simulink model "hcu_main_dspace"  (Simulink 8.2)
settings: Solver=FixedStepDiscrete  StartTime=0.0  StopTime=Inf  FixedStep=0.005  RelTol=1e-3
PostLoadFcn:
  | , if any(exist('dsrtsu_mdlpostloadfcn', 'file') == [2, 3, 6]), try dsrtsu_mdlpostloadfcn('Execute', bdroot); catch fprintf('Error in PostLoadFcn (dsrtsu_mdlpostloadfcn) for model "%s":\n %s\n', bdroot, lasterr); end, end,
values from neighbouring files (symbols this model uses):
  C_TASK_5MS_S = (	C_TICK_TIME_S      	)    [hcu_local_hdr.m]
  ENUM_GEARPOSN_1ST = uint8(  1  )    [hcu_local_hdr.m]
  ENUM_GEARPOSN_2ND = uint8(  2  )    [hcu_local_hdr.m]
  ENUM_GEARPOSN_3RD = uint8(  3  )    [hcu_local_hdr.m]
  ENUM_GEARPOSN_4TH = uint8(  4  )    [hcu_local_hdr.m]
  ENUM_GEARPOSN_5TH = uint8(  5  )    [hcu_local_hdr.m]
  ENUM_GEARPOSN_6TH = uint8(  6  )    [hcu_local_hdr.m]
  ENUM_GEARPOSN_R = uint8(  7  )    [hcu_local_hdr.m]
undefined symbols (not defined in the file or in its folder): rticanmm_blockfcn, rticanmm_initfcn
libraries: rtimmsu_dsrtlib x3, simulink x2, hal x2, app x1, rtiethernetudplib x1, inp x1, outp x1, hcu_lib x1
(part 3 of 4)

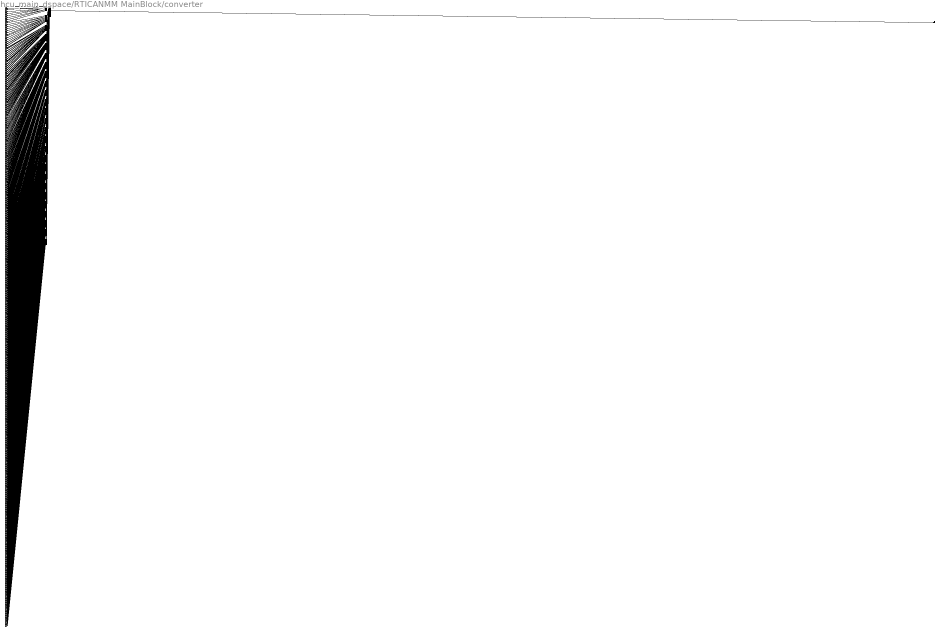
== system hcu_main_dspace/RTICANMM MainBlock/converter ==
  in_1 : Inport
  in_2 : Inport  Port=2
  in_3 : Inport  Port=3
  in_4 : Inport  Port=4
  in_5 : Inport  Port=5
  in_6 : Inport  Port=6
  in_7 : Inport  Port=7
  in_8 : Inport  Port=8
  in_9 : Inport  Port=9
  in_10 : Inport  Port=10
  in_11 : Inport  Port=11
  in_12 : Inport  Port=12
  in_13 : Inport  Port=13
  in_14 : Inport  Port=14
  in_15 : Inport  Port=15
  in_16 : Inport  Port=16
  in_17 : Inport  Port=17
  in_18 : Inport  Port=18
  in_19 : Inport  Port=19
  in_20 : Inport  Port=20
  in_21 : Inport  Port=21
  in_22 : Inport  Port=22
  in_23 : Inport  Port=23
  in_24 : Inport  Port=24
  in_25 : Inport  Port=25
  in_26 : Inport  Port=26
  in_27 : Inport  Port=27
  in_28 : Inport  Port=28
  in_29 : Inport  Port=29
  in_30 : Inport  Port=30
  in_31 : Inport  Port=31
  in_32 : Inport  Port=32
  in_33 : Inport  Port=33
  in_34 : Inport  Port=34
  in_35 : Inport  Port=35
  in_36 : Inport  Port=36
  in_37 : Inport  Port=37
  in_38 : Inport  Port=38
  in_39 : Inport  Port=39
  in_40 : Inport  Port=40
  in_41 : Inport  Port=41
  in_42 : Inport  Port=42
  in_43 : Inport  Port=43
  in_44 : Inport  Port=44
  in_45 : Inport  Port=45
  in_46 : Inport  Port=46
  in_47 : Inport  Port=47
  in_48 : Inport  Port=48
  in_49 : Inport  Port=49
  in_50 : Inport  Port=50
  in_51 : Inport  Port=51
  in_52 : Inport  Port=52
  in_53 : Inport  Port=53
  in_54 : Inport  Port=54
  in_55 : Inport  Port=55
  in_56 : Inport  Port=56
  in_57 : Inport  Port=57
  in_58 : Inport  Port=58
  in_59 : Inport  Port=59
  in_60 : Inport  Port=60
  in_61 : Inport  Port=61
  in_62 : Inport  Port=62
  in_63 : Inport  Port=63
  in_64 : Inport  Port=64
  in_65 : Inport  Port=65
  in_66 : Inport  Port=66
  in_67 : Inport  Port=67
  in_68 : Inport  Port=68
  in_69 : Inport  Port=69
  in_70 : Inport  Port=70
  in_71 : Inport  Port=71
  in_72 : Inport  Port=72
  in_73 : Inport  Port=73
  in_74 : Inport  Port=74
  in_75 : Inport  Port=75
  in_76 : Inport  Port=76
  in_77 : Inport  Port=77
  in_78 : Inport  Port=78
  in_79 : Inport  Port=79
  in_80 : Inport  Port=80
  in_81 : Inport  Port=81
  in_82 : Inport  Port=82
  in_83 : Inport  Port=83
  in_84 : Inport  Port=84
  in_85 : Inport  Port=85
  in_86 : Inport  Port=86
  in_87 : Inport  Port=87
  in_88 : Inport  Port=88
  in_89 : Inport  Port=89
  in_90 : Inport  Port=90
  in_91 : Inport  Port=91
  in_92 : Inport  Port=92
  in_93 : Inport  Port=93
  in_94 : Inport  Port=94
  in_95 : Inport  Port=95
  in_96 : Inport  Port=96
  in_97 : Inport  Port=97
  in_98 : Inport  Port=98
  in_99 : Inport  Port=99
  in_100 : Inport  Port=100
  in_101 : Inport  Port=101
  in_102 : Inport  Port=102
  in_103 : Inport  Port=103
  in_104 : Inport  Port=104
  in_105 : Inport  Port=105
  in_106 : Inport  Port=106
  in_107 : Inport  Port=107
  in_108 : Inport  Port=108
  in_109 : Inport  Port=109
  in_110 : Inport  Port=110
  in_111 : Inport  Port=111
  in_112 : Inport  Port=112
  in_113 : Inport  Port=113
  in_114 : Inport  Port=114
  in_115 : Inport  Port=115
  in_116 : Inport  Port=116
  in_117 : Inport  Port=117
  in_118 : Inport  Port=118
  in_119 : Inport  Port=119
  in_120 : Inport  Port=120
  in_121 : Inport  Port=121
  in_122 : Inport  Port=122
  in_123 : Inport  Port=123
  in_124 : Inport  Port=124
  in_125 : Inport  Port=125
  in_126 : Inport  Port=126
  in_127 : Inport  Port=127
  in_128 : Inport  Port=128
  in_129 : Inport  Port=129
  in_130 : Inport  Port=130
  in_131 : Inport  Port=131
  in_132 : Inport  Port=132
  in_133 : Inport  Port=133
  in_134 : Inport  Port=134
  in_135 : Inport  Port=135
  in_136 : Inport  Port=136
  in_137 : Inport  Port=137
  in_138 : Inport  Port=138
  in_139 : Inport  Port=139
  in_140 : Inport  Port=140
  in_141 : Inport  Port=141
  in_142 : Inport  Port=142
  in_143 : Inport  Port=143
  in_144 : Inport  Port=144
  in_145 : Inport  Port=145
  in_146 : Inport  Port=146
  in_147 : Inport  Port=147
  in_148 : Inport  Port=148
  in_149 : Inport  Port=149
  in_150 : Inport  Port=150
  in_151 : Inport  Port=151
  in_152 : Inport  Port=152
  in_153 : Inport  Port=153
  in_154 : Inport  Port=154
  in_155 : Inport  Port=155
  in_156 : Inport  Port=156
  in_157 : Inport  Port=157
  in_158 : Inport  Port=158
  in_159 : Inport  Port=159
  in_160 : Inport  Port=160
  in_161 : Inport  Port=161
  in_162 : Inport  Port=162
  in_163 : Inport  Port=163
  in_164 : Inport  Port=164
  in_165 : Inport  Port=165
  in_166 : Inport  Port=166
  in_167 : Inport  Port=167
  in_168 : Inport  Port=168
  in_169 : Inport  Port=169
  in_170 : Inport  Port=170
  in_171 : Inport  Port=171
  in_172 : Inport  Port=172
  in_173 : Inport  Port=173
  in_174 : Inport  Port=174
  in_175 : Inport  Port=175
  in_176 : Inport  Port=176
  in_177 : Inport  Port=177
  in_178 : Inport  Port=178
  in_179 : Inport  Port=179
  in_180 : Inport  Port=180
  in_181 : Inport  Port=181
  in_182 : Inport  Port=182
  in_183 : Inport  Port=183
  in_184 : Inport  Port=184
  in_185 : Inport  Port=185
  in_186 : Inport  Port=186
  in_187 : Inport  Port=187
  in_188 : Inport  Port=188
  in_189 : Inport  Port=189
  in_190 : Inport  Port=190
  in_191 : Inport  Port=191
  in_192 : Inport  Port=192
  in_193 : Inport  Port=193
  in_194 : Inport  Port=194
  in_195 : Inport  Port=195
  in_196 : Inport  Port=196
  in_197 : Inport  Port=197
  in_198 : Inport  Port=198
  in_199 : Inport  Port=199
  in_200 : Inport  Port=200
  in_201 : Inport  Port=201
  in_202 : Inport  Port=202
  in_203 : Inport  Port=203
  in_204 : Inport  Port=204
  in_205 : Inport  Port=205
  in_206 : Inport  Port=206
  in_207 : Inport  Port=207
  in_208 : Inport  Port=208
  in_209 : Inport  Port=209
  in_210 : Inport  Port=210
  in_211 : Inport  Port=211
  in_212 : Inport  Port=212
  in_213 : Inport  Port=213
  in_214 : Inport  Port=214
  in_215 : Inport  Port=215
  in_216 : Inport  Port=216
  in_217 : Inport  Port=217
  in_218 : Inport  Port=218
  in_219 : Inport  Port=219
  in_220 : Inport  Port=220
  in_221 : Inport  Port=221
  in_222 : Inport  Port=222
  in_223 : Inport  Port=223
  in_224 : Inport  Port=224
  in_225 : Inport  Port=225
  in_226 : Inport  Port=226
  in_227 : Inport  Port=227
  in_228 : Inport  Port=228
  in_229 : Inport  Port=229
  in_230 : Inport  Port=230
  in_231 : Inport  Port=231
  in_232 : Inport  Port=232
  in_233 : Inport  Port=233
  in_234 : Inport  Port=234
  in_235 : Inport  Port=235
  in_236 : Inport  Port=236
  in_237 : Inport  Port=237
  in_238 : Inport  Port=238
  in_239 : Inport  Port=239
  in_240 : Inport  Port=240
  in_241 : Inport  Port=241
  in_242 : Inport  Port=242
  in_243 : Inport  Port=243
  in_244 : Inport  Port=244
  in_245 : Inport  Port=245
  in_246 : Inport  Port=246
  in_247 : Inport  Port=247
  in_248 : Inport  Port=248
  in_249 : Inport  Port=249
  in_250 : Inport  Port=250
  in_251 : Inport  Port=251
  in_252 : Inport  Port=252
  in_253 : Inport  Port=253
  in_254 : Inport  Port=254
  in_255 : Inport  Port=255
  in_256 : Inport  Port=256
  in_257 : Inport  Port=257
  in_258 : Inport  Port=258
  in_259 : Inport  Port=259
  in_260 : Inport  Port=260
  in_261 : Inport  Port=261
  in_262 : Inport  Port=262
  in_263 : Inport  Port=263
  in_264 : Inport  Port=264
  in_265 : Inport  Port=265
  in_266 : Inport  Port=266
  in_267 : Inport  Port=267
  in_268 : Inport  Port=268
  in_269 : Inport  Port=269
  in_270 : Inport  Port=270
  in_271 : Inport  Port=271
  in_272 : Inport  Port=272
  in_273 : Inport  Port=273
  in_274 : Inport  Port=274
  in_275 : Inport  Port=275
  in_276 : Inport  Port=276
  in_277 : Inport  Port=277
  in_278 : Inport  Port=278
  in_279 : Inport  Port=279
  in_280 : Inport  Port=280
  in_281 : Inport  Port=281
  in_282 : Inport  Port=282
  in_283 : Inport  Port=283
  in_284 : Inport  Port=284
  in_285 : Inport  Port=285
  in_286 : Inport  Port=286
  in_287 : Inport  Port=287
  in_288 : Inport  Port=288
  in_289 : Inport  Port=289
  in_290 : Inport  Port=290
  in_291 : Inport  Port=291
  in_292 : Inport  Port=292
  in_293 : Inport  Port=293
  in_294 : Inport  Port=294
  in_295 : Inport  Port=295
  in_296 : Inport  Port=296
  in_297 : Inport  Port=297
  in_298 : Inport  Port=298
  in_299 : Inport  Port=299
  in_300 : Inport  Port=300
  in_301 : Inport  Port=301
  in_302 : Inport  Port=302
  in_303 : Inport  Port=303
  in_304 : Inport  Port=304
  in_305 : Inport  Port=305
  in_306 : Inport  Port=306
  in_307 : Inport  Port=307
  in_308 : Inport  Port=308
  in_309 : Inport  Port=309
  in_310 : Inport  Port=310
  in_311 : Inport  Port=311
  in_312 : Inport  Port=312
  in_313 : Inport  Port=313
  in_314 : Inport  Port=314
  in_315 : Inport  Port=315
  in_316 : Inport  Port=316
  in_317 : Inport  Port=317
  in_318 : Inport  Port=318
  in_319 : Inport  Port=319
  in_320 : Inport  Port=320
  in_321 : Inport  Port=321
  in_322 : Inport  Port=322
  in_323 : Inport  Port=323
  in_324 : Inport  Port=324
  in_325 : Inport  Port=325
  in_326 : Inport  Port=326
  in_327 : Inport  Port=327
  in_328 : Inport  Port=328
  in_329 : Inport  Port=329
  in_330 : Inport  Port=330
  in_331 : Inport  Port=331
  in_332 : Inport  Port=332
  in_333 : Inport  Port=333
  in_334 : Inport  Port=334
  Lane_Details : BusCreator  Inputs=9
  Mux : BusCreator  Inputs=26
  RTICANMMCaptureMessage_{1..25} (25 alike) : BusCreator  Inputs=13
  out : Outport
  wires:
  in_1/1 -> Lane_Details/1  "Left_Guard_Rail"
  Lane_Details/1 -> Mux/1  "Lane_Details"
  in_2/1 -> Lane_Details/2  "Right_Guard_Rail"
  in_3/1 -> Lane_Details/3  "construction_area"
  in_4/1 -> Lane_Details/4  "Right_LDW_Availability"
  in_5/1 -> Lane_Details/5  "Left_LDW_Availability"
  in_6/1 -> Lane_Details/6  "Yaw_Angle"
  in_7/1 -> Lane_Details/7  "Pitch_Angle"
  in_8/1 -> Lane_Details/8  "Number_of_Lanes"
  in_9/1 -> Lane_Details/9  "Position_in_Lanes"
  in_10/1 -> RTICANMMCaptureMessage_1/1  "Status"
  RTICANMMCaptureMessage_1/1 -> Mux/2  "RTICANMMCaptureMessage_1"
  in_11/1 -> RTICANMMCaptureMessage_1/2  "Time"
  in_12/1 -> RTICANMMCaptureMessage_1/3  "ID"
  in_13/1 -> RTICANMMCaptureMessage_1/4  "MessageIDFormat"
  in_14/1 -> RTICANMMCaptureMessage_1/5  "Length"
  in_15/1 -> RTICANMMCaptureMessage_1/6  "RAW_Byte_1"
  in_16/1 -> RTICANMMCaptureMessage_1/7  "RAW_Byte_2"
  in_17/1 -> RTICANMMCaptureMessage_1/8  "RAW_Byte_3"
  in_18/1 -> RTICANMMCaptureMessage_1/9  "RAW_Byte_4"
  in_19/1 -> RTICANMMCaptureMessage_1/10  "RAW_Byte_5"
  in_20/1 -> RTICANMMCaptureMessage_1/11  "RAW_Byte_6"
  in_21/1 -> RTICANMMCaptureMessage_1/12  "RAW_Byte_7"
  in_22/1 -> RTICANMMCaptureMessage_1/13  "RAW_Byte_8"
  in_23/1 -> RTICANMMCaptureMessage_2/1  "Status"
  RTICANMMCaptureMessage_2/1 -> Mux/3  "RTICANMMCaptureMessage_2"
  in_24/1 -> RTICANMMCaptureMessage_2/2  "Time"
  in_25/1 -> RTICANMMCaptureMessage_2/3  "ID"
  in_26/1 -> RTICANMMCaptureMessage_2/4  "MessageIDFormat"
  in_27/1 -> RTICANMMCaptureMessage_2/5  "Length"
  in_28/1 -> RTICANMMCaptureMessage_2/6  "RAW_Byte_1"
  in_29/1 -> RTICANMMCaptureMessage_2/7  "RAW_Byte_2"
  in_30/1 -> RTICANMMCaptureMessage_2/8  "RAW_Byte_3"
  in_31/1 -> RTICANMMCaptureMessage_2/9  "RAW_Byte_4"
  in_32/1 -> RTICANMMCaptureMessage_2/10  "RAW_Byte_5"
  in_33/1 -> RTICANMMCaptureMessage_2/11  "RAW_Byte_6"
  in_34/1 -> RTICANMMCaptureMessage_2/12  "RAW_Byte_7"
  in_35/1 -> RTICANMMCaptureMessage_2/13  "RAW_Byte_8"
  in_36/1 -> RTICANMMCaptureMessage_3/1  "Status"
  RTICANMMCaptureMessage_3/1 -> Mux/4  "RTICANMMCaptureMessage_3"
  in_37/1 -> RTICANMMCaptureMessage_3/2  "Time"
  in_38/1 -> RTICANMMCaptureMessage_3/3  "ID"
  in_39/1 -> RTICANMMCaptureMessage_3/4  "MessageIDFormat"
  in_40/1 -> RTICANMMCaptureMessage_3/5  "Length"
  in_41/1 -> RTICANMMCaptureMessage_3/6  "RAW_Byte_1"
  in_42/1 -> RTICANMMCaptureMessage_3/7  "RAW_Byte_2"
  in_43/1 -> RTICANMMCaptureMessage_3/8  "RAW_Byte_3"
  in_44/1 -> RTICANMMCaptureMessage_3/9  "RAW_Byte_4"
  in_45/1 -> RTICANMMCaptureMessage_3/10  "RAW_Byte_5"
  in_46/1 -> RTICANMMCaptureMessage_3/11  "RAW_Byte_6"
  in_47/1 -> RTICANMMCaptureMessage_3/12  "RAW_Byte_7"
  in_48/1 -> RTICANMMCaptureMessage_3/13  "RAW_Byte_8"
  in_49/1 -> RTICANMMCaptureMessage_4/1  "Status"
  RTICANMMCaptureMessage_4/1 -> Mux/5  "RTICANMMCaptureMessage_4"
  in_50/1 -> RTICANMMCaptureMessage_4/2  "Time"
  in_51/1 -> RTICANMMCaptureMessage_4/3  "ID"
  in_52/1 -> RTICANMMCaptureMessage_4/4  "MessageIDFormat"
  in_53/1 -> RTICANMMCaptureMessage_4/5  "Length"
  in_54/1 -> RTICANMMCaptureMessage_4/6  "RAW_Byte_1"
  in_55/1 -> RTICANMMCaptureMessage_4/7  "RAW_Byte_2"
  in_56/1 -> RTICANMMCaptureMessage_4/8  "RAW_Byte_3"
  in_57/1 -> RTICANMMCaptureMessage_4/9  "RAW_Byte_4"
  in_58/1 -> RTICANMMCaptureMessage_4/10  "RAW_Byte_5"
  in_59/1 -> RTICANMMCaptureMessage_4/11  "RAW_Byte_6"
  in_60/1 -> RTICANMMCaptureMessage_4/12  "RAW_Byte_7"
  in_61/1 -> RTICANMMCaptureMessage_4/13  "RAW_Byte_8"
  in_62/1 -> RTICANMMCaptureMessage_5/1  "Status"
  RTICANMMCaptureMessage_5/1 -> Mux/6  "RTICANMMCaptureMessage_5"
  in_63/1 -> RTICANMMCaptureMessage_5/2  "Time"
  in_64/1 -> RTICANMMCaptureMessage_5/3  "ID"
  in_65/1 -> RTICANMMCaptureMessage_5/4  "MessageIDFormat"
  in_66/1 -> RTICANMMCaptureMessage_5/5  "Length"
  in_67/1 -> RTICANMMCaptureMessage_5/6  "RAW_Byte_1"
  in_68/1 -> RTICANMMCaptureMessage_5/7  "RAW_Byte_2"
  in_69/1 -> RTICANMMCaptureMessage_5/8  "RAW_Byte_3"
  in_70/1 -> RTICANMMCaptureMessage_5/9  "RAW_Byte_4"
  in_71/1 -> RTICANMMCaptureMessage_5/10  "RAW_Byte_5"
  in_72/1 -> RTICANMMCaptureMessage_5/11  "RAW_Byte_6"
  in_73/1 -> RTICANMMCaptureMessage_5/12  "RAW_Byte_7"
  in_74/1 -> RTICANMMCaptureMessage_5/13  "RAW_Byte_8"
  in_75/1 -> RTICANMMCaptureMessage_6/1  "Status"
  RTICANMMCaptureMessage_6/1 -> Mux/7  "RTICANMMCaptureMessage_6"
  in_76/1 -> RTICANMMCaptureMessage_6/2  "Time"
  in_77/1 -> RTICANMMCaptureMessage_6/3  "ID"
  in_78/1 -> RTICANMMCaptureMessage_6/4  "MessageIDFormat"
  in_79/1 -> RTICANMMCaptureMessage_6/5  "Length"
  in_80/1 -> RTICANMMCaptureMessage_6/6  "RAW_Byte_1"
  in_81/1 -> RTICANMMCaptureMessage_6/7  "RAW_Byte_2"
  in_82/1 -> RTICANMMCaptureMessage_6/8  "RAW_Byte_3"
  in_83/1 -> RTICANMMCaptureMessage_6/9  "RAW_Byte_4"
  in_84/1 -> RTICANMMCaptureMessage_6/10  "RAW_Byte_5"
  in_85/1 -> RTICANMMCaptureMessage_6/11  "RAW_Byte_6"
  in_86/1 -> RTICANMMCaptureMessage_6/12  "RAW_Byte_7"
  in_87/1 -> RTICANMMCaptureMessage_6/13  "RAW_Byte_8"
  in_88/1 -> RTICANMMCaptureMessage_7/1  "Status"
  RTICANMMCaptureMessage_7/1 -> Mux/8  "RTICANMMCaptureMessage_7"
  in_89/1 -> RTICANMMCaptureMessage_7/2  "Time"
  in_90/1 -> RTICANMMCaptureMessage_7/3  "ID"
  in_91/1 -> RTICANMMCaptureMessage_7/4  "MessageIDFormat"
  in_92/1 -> RTICANMMCaptureMessage_7/5  "Length"
  in_93/1 -> RTICANMMCaptureMessage_7/6  "RAW_Byte_1"
  in_94/1 -> RTICANMMCaptureMessage_7/7  "RAW_Byte_2"
  in_95/1 -> RTICANMMCaptureMessage_7/8  "RAW_Byte_3"
  in_96/1 -> RTICANMMCaptureMessage_7/9  "RAW_Byte_4"
  in_97/1 -> RTICANMMCaptureMessage_7/10  "RAW_Byte_5"
  in_98/1 -> RTICANMMCaptureMessage_7/11  "RAW_Byte_6"
  in_99/1 -> RTICANMMCaptureMessage_7/12  "RAW_Byte_7"
  in_100/1 -> RTICANMMCaptureMessage_7/13  "RAW_Byte_8"
  in_101/1 -> RTICANMMCaptureMessage_8/1  "Status"
  RTICANMMCaptureMessage_8/1 -> Mux/9  "RTICANMMCaptureMessage_8"
  in_102/1 -> RTICANMMCaptureMessage_8/2  "Time"
  in_103/1 -> RTICANMMCaptureMessage_8/3  "ID"
  in_104/1 -> RTICANMMCaptureMessage_8/4  "MessageIDFormat"
  in_105/1 -> RTICANMMCaptureMessage_8/5  "Length"
  in_106/1 -> RTICANMMCaptureMessage_8/6  "RAW_Byte_1"
  in_107/1 -> RTICANMMCaptureMessage_8/7  "RAW_Byte_2"
  in_108/1 -> RTICANMMCaptureMessage_8/8  "RAW_Byte_3"
  in_109/1 -> RTICANMMCaptureMessage_8/9  "RAW_Byte_4"
  in_110/1 -> RTICANMMCaptureMessage_8/10  "RAW_Byte_5"
  in_111/1 -> RTICANMMCaptureMessage_8/11  "RAW_Byte_6"
  in_112/1 -> RTICANMMCaptureMessage_8/12  "RAW_Byte_7"
  in_113/1 -> RTICANMMCaptureMessage_8/13  "RAW_Byte_8"
  in_114/1 -> RTICANMMCaptureMessage_9/1  "Status"
  RTICANMMCaptureMessage_9/1 -> Mux/10  "RTICANMMCaptureMessage_9"
  in_115/1 -> RTICANMMCaptureMessage_9/2  "Time"
  in_116/1 -> RTICANMMCaptureMessage_9/3  "ID"
  in_117/1 -> RTICANMMCaptureMessage_9/4  "MessageIDFormat"
  in_118/1 -> RTICANMMCaptureMessage_9/5  "Length"
  in_119/1 -> RTICANMMCaptureMessage_9/6  "RAW_Byte_1"
  in_120/1 -> RTICANMMCaptureMessage_9/7  "RAW_Byte_2"
  in_121/1 -> RTICANMMCaptureMessage_9/8  "RAW_Byte_3"
  in_122/1 -> RTICANMMCaptureMessage_9/9  "RAW_Byte_4"
  in_123/1 -> RTICANMMCaptureMessage_9/10  "RAW_Byte_5"
  in_124/1 -> RTICANMMCaptureMessage_9/11  "RAW_Byte_6"
  in_125/1 -> RTICANMMCaptureMessage_9/12  "RAW_Byte_7"
  in_126/1 -> RTICANMMCaptureMessage_9/13  "RAW_Byte_8"
  in_127/1 -> RTICANMMCaptureMessage_10/1  "Status"
  RTICANMMCaptureMessage_10/1 -> Mux/11  "RTICANMMCaptureMessage_10"
  in_128/1 -> RTICANMMCaptureMessage_10/2  "Time"
  in_129/1 -> RTICANMMCaptureMessage_10/3  "ID"
  in_130/1 -> RTICANMMCaptureMessage_10/4  "MessageIDFormat"
  in_131/1 -> RTICANMMCaptureMessage_10/5  "Length"
  in_132/1 -> RTICANMMCaptureMessage_10/6  "RAW_Byte_1"
  in_133/1 -> RTICANMMCaptureMessage_10/7  "RAW_Byte_2"
  in_134/1 -> RTICANMMCaptureMessage_10/8  "RAW_Byte_3"
  in_135/1 -> RTICANMMCaptureMessage_10/9  "RAW_Byte_4"
  in_136/1 -> RTICANMMCaptureMessage_10/10  "RAW_Byte_5"
  in_137/1 -> RTICANMMCaptureMessage_10/11  "RAW_Byte_6"
  in_138/1 -> RTICANMMCaptureMessage_10/12  "RAW_Byte_7"
  in_139/1 -> RTICANMMCaptureMessage_10/13  "RAW_Byte_8"
  in_140/1 -> RTICANMMCaptureMessage_11/1  "Status"
  RTICANMMCaptureMessage_11/1 -> Mux/12  "RTICANMMCaptureMessage_11"
  in_141/1 -> RTICANMMCaptureMessage_11/2  "Time"
  in_142/1 -> RTICANMMCaptureMessage_11/3  "ID"
  in_143/1 -> RTICANMMCaptureMessage_11/4  "MessageIDFormat"
  in_144/1 -> RTICANMMCaptureMessage_11/5  "Length"
  in_145/1 -> RTICANMMCaptureMessage_11/6  "RAW_Byte_1"
  in_146/1 -> RTICANMMCaptureMessage_11/7  "RAW_Byte_2"
  in_147/1 -> RTICANMMCaptureMessage_11/8  "RAW_Byte_3"
  in_148/1 -> RTICANMMCaptureMessage_11/9  "RAW_Byte_4"
  in_149/1 -> RTICANMMCaptureMessage_11/10  "RAW_Byte_5"
  in_150/1 -> RTICANMMCaptureMessage_11/11  "RAW_Byte_6"
  in_151/1 -> RTICANMMCaptureMessage_11/12  "RAW_Byte_7"
  in_152/1 -> RTICANMMCaptureMessage_11/13  "RAW_Byte_8"
  in_153/1 -> RTICANMMCaptureMessage_12/1  "Status"
  RTICANMMCaptureMessage_12/1 -> Mux/13  "RTICANMMCaptureMessage_12"
  in_154/1 -> RTICANMMCaptureMessage_12/2  "Time"
  in_155/1 -> RTICANMMCaptureMessage_12/3  "ID"
  in_156/1 -> RTICANMMCaptureMessage_12/4  "MessageIDFormat"
  in_157/1 -> RTICANMMCaptureMessage_12/5  "Length"
  in_158/1 -> RTICANMMCaptureMessage_12/6  "RAW_Byte_1"
  in_159/1 -> RTICANMMCaptureMessage_12/7  "RAW_Byte_2"
  in_160/1 -> RTICANMMCaptureMessage_12/8  "RAW_Byte_3"
  in_161/1 -> RTICANMMCaptureMessage_12/9  "RAW_Byte_4"
  in_162/1 -> RTICANMMCaptureMessage_12/10  "RAW_Byte_5"
  in_163/1 -> RTICANMMCaptureMessage_12/11  "RAW_Byte_6"
  in_164/1 -> RTICANMMCaptureMessage_12/12  "RAW_Byte_7"
  in_165/1 -> RTICANMMCaptureMessage_12/13  "RAW_Byte_8"
  in_166/1 -> RTICANMMCaptureMessage_13/1  "Status"
  RTICANMMCaptureMessage_13/1 -> Mux/14  "RTICANMMCaptureMessage_13"
  in_167/1 -> RTICANMMCaptureMessage_13/2  "Time"
  in_168/1 -> RTICANMMCaptureMessage_13/3  "ID"
  in_169/1 -> RTICANMMCaptureMessage_13/4  "MessageIDFormat"
  in_170/1 -> RTICANMMCaptureMessage_13/5  "Length"
  in_171/1 -> RTICANMMCaptureMessage_13/6  "RAW_Byte_1"
  in_172/1 -> RTICANMMCaptureMessage_13/7  "RAW_Byte_2"
  in_173/1 -> RTICANMMCaptureMessage_13/8  "RAW_Byte_3"
  in_174/1 -> RTICANMMCaptureMessage_13/9  "RAW_Byte_4"
  in_175/1 -> RTICANMMCaptureMessage_13/10  "RAW_Byte_5"
  in_176/1 -> RTICANMMCaptureMessage_13/11  "RAW_Byte_6"
  in_177/1 -> RTICANMMCaptureMessage_13/12  "RAW_Byte_7"
  in_178/1 -> RTICANMMCaptureMessage_13/13  "RAW_Byte_8"
  in_179/1 -> RTICANMMCaptureMessage_14/1  "Status"
  RTICANMMCaptureMessage_14/1 -> Mux/15  "RTICANMMCaptureMessage_14"
  in_180/1 -> RTICANMMCaptureMessage_14/2  "Time"
  in_181/1 -> RTICANMMCaptureMessage_14/3  "ID"
  in_182/1 -> RTICANMMCaptureMessage_14/4  "MessageIDFormat"
  in_183/1 -> RTICANMMCaptureMessage_14/5  "Length"
  in_184/1 -> RTICANMMCaptureMessage_14/6  "RAW_Byte_1"
  in_185/1 -> RTICANMMCaptureMessage_14/7  "RAW_Byte_2"
  in_186/1 -> RTICANMMCaptureMessage_14/8  "RAW_Byte_3"
  in_187/1 -> RTICANMMCaptureMessage_14/9  "RAW_Byte_4"
  in_188/1 -> RTICANMMCaptureMessage_14/10  "RAW_Byte_5"
  in_189/1 -> RTICANMMCaptureMessage_14/11  "RAW_Byte_6"
  in_190/1 -> RTICANMMCaptureMessage_14/12  "RAW_Byte_7"
  in_191/1 -> RTICANMMCaptureMessage_14/13  "RAW_Byte_8"
  in_192/1 -> RTICANMMCaptureMessage_15/1  "Status"
  RTICANMMCaptureMessage_15/1 -> Mux/16  "RTICANMMCaptureMessage_15"
  in_193/1 -> RTICANMMCaptureMessage_15/2  "Time"
  in_194/1 -> RTICANMMCaptureMessage_15/3  "ID"
  in_195/1 -> RTICANMMCaptureMessage_15/4  "MessageIDFormat"
  in_196/1 -> RTICANMMCaptureMessage_15/5  "Length"
  in_197/1 -> RTICANMMCaptureMessage_15/6  "RAW_Byte_1"
  in_198/1 -> RTICANMMCaptureMessage_15/7  "RAW_Byte_2"
  in_199/1 -> RTICANMMCaptureMessage_15/8  "RAW_Byte_3"
  in_200/1 -> RTICANMMCaptureMessage_15/9  "RAW_Byte_4"
  in_201/1 -> RTICANMMCaptureMessage_15/10  "RAW_Byte_5"
  in_202/1 -> RTICANMMCaptureMessage_15/11  "RAW_Byte_6"
  in_203/1 -> RTICANMMCaptureMessage_15/12  "RAW_Byte_7"
  in_204/1 -> RTICANMMCaptureMessage_15/13  "RAW_Byte_8"
  in_205/1 -> RTICANMMCaptureMessage_16/1  "Status"
  RTICANMMCaptureMessage_16/1 -> Mux/17  "RTICANMMCaptureMessage_16"
  in_206/1 -> RTICANMMCaptureMessage_16/2  "Time"
  in_207/1 -> RTICANMMCaptureMessage_16/3  "ID"
  in_208/1 -> RTICANMMCaptureMessage_16/4  "MessageIDFormat"
  in_209/1 -> RTICANMMCaptureMessage_16/5  "Length"
  in_210/1 -> RTICANMMCaptureMessage_16/6  "RAW_Byte_1"
  in_211/1 -> RTICANMMCaptureMessage_16/7  "RAW_Byte_2"
  in_212/1 -> RTICANMMCaptureMessage_16/8  "RAW_Byte_3"
  in_213/1 -> RTICANMMCaptureMessage_16/9  "RAW_Byte_4"
  in_214/1 -> RTICANMMCaptureMessage_16/10  "RAW_Byte_5"
  in_215/1 -> RTICANMMCaptureMessage_16/11  "RAW_Byte_6"
  in_216/1 -> RTICANMMCaptureMessage_16/12  "RAW_Byte_7"
  in_217/1 -> RTICANMMCaptureMessage_16/13  "RAW_Byte_8"
  in_218/1 -> RTICANMMCaptureMessage_17/1  "Status"
  RTICANMMCaptureMessage_17/1 -> Mux/18  "RTICANMMCaptureMessage_17"
  in_219/1 -> RTICANMMCaptureMessage_17/2  "Time"
  in_220/1 -> RTICANMMCaptureMessage_17/3  "ID"
  in_221/1 -> RTICANMMCaptureMessage_17/4  "MessageIDFormat"
  in_222/1 -> RTICANMMCaptureMessage_17/5  "Length"
  in_223/1 -> RTICANMMCaptureMessage_17/6  "RAW_Byte_1"
  in_224/1 -> RTICANMMCaptureMessage_17/7  "RAW_Byte_2"
  in_225/1 -> RTICANMMCaptureMessage_17/8  "RAW_Byte_3"
  in_226/1 -> RTICANMMCaptureMessage_17/9  "RAW_Byte_4"
  in_227/1 -> RTICANMMCaptureMessage_17/10  "RAW_Byte_5"
  in_228/1 -> RTICANMMCaptureMessage_17/11  "RAW_Byte_6"
  in_229/1 -> RTICANMMCaptureMessage_17/12  "RAW_Byte_7"
  in_230/1 -> RTICANMMCaptureMessage_17/13  "RAW_Byte_8"
  in_231/1 -> RTICANMMCaptureMessage_18/1  "Status"
  RTICANMMCaptureMessage_18/1 -> Mux/19  "RTICANMMCaptureMessage_18"
  in_232/1 -> RTICANMMCaptureMessage_18/2  "Time"
  in_233/1 -> RTICANMMCaptureMessage_18/3  "ID"
  in_234/1 -> RTICANMMCaptureMessage_18/4  "MessageIDFormat"
  in_235/1 -> RTICANMMCaptureMessage_18/5  "Length"
  in_236/1 -> RTICANMMCaptureMessage_18/6  "RAW_Byte_1"
  in_237/1 -> RTICANMMCaptureMessage_18/7  "RAW_Byte_2"
  in_238/1 -> RTICANMMCaptureMessage_18/8  "RAW_Byte_3"
  in_239/1 -> RTICANMMCaptureMessage_18/9  "RAW_Byte_4"
  in_240/1 -> RTICANMMCaptureMessage_18/10  "RAW_Byte_5"
  in_241/1 -> RTICANMMCaptureMessage_18/11  "RAW_Byte_6"
  in_242/1 -> RTICANMMCaptureMessage_18/12  "RAW_Byte_7"
  in_243/1 -> RTICANMMCaptureMessage_18/13  "RAW_Byte_8"
  in_244/1 -> RTICANMMCaptureMessage_19/1  "Status"
  RTICANMMCaptureMessage_19/1 -> Mux/20  "RTICANMMCaptureMessage_19"
  in_245/1 -> RTICANMMCaptureMessage_19/2  "Time"
  in_246/1 -> RTICANMMCaptureMessage_19/3  "ID"
  in_247/1 -> RTICANMMCaptureMessage_19/4  "MessageIDFormat"
  in_248/1 -> RTICANMMCaptureMessage_19/5  "Length"
  in_249/1 -> RTICANMMCaptureMessage_19/6  "RAW_Byte_1"
  in_250/1 -> RTICANMMCaptureMessage_19/7  "RAW_Byte_2"
  in_251/1 -> RTICANMMCaptureMessage_19/8  "RAW_Byte_3"
  in_252/1 -> RTICANMMCaptureMessage_19/9  "RAW_Byte_4"
  in_253/1 -> RTICANMMCaptureMessage_19/10  "RAW_Byte_5"
  in_254/1 -> RTICANMMCaptureMessage_19/11  "RAW_Byte_6"
  in_255/1 -> RTICANMMCaptureMessage_19/12  "RAW_Byte_7"
  in_256/1 -> RTICANMMCaptureMessage_19/13  "RAW_Byte_8"
  in_257/1 -> RTICANMMCaptureMessage_20/1  "Status"
  RTICANMMCaptureMessage_20/1 -> Mux/21  "RTICANMMCaptureMessage_20"
  in_258/1 -> RTICANMMCaptureMessage_20/2  "Time"
  in_259/1 -> RTICANMMCaptureMessage_20/3  "ID"
  in_260/1 -> RTICANMMCaptureMessage_20/4  "MessageIDFormat"
  in_261/1 -> RTICANMMCaptureMessage_20/5  "Length"
  in_262/1 -> RTICANMMCaptureMessage_20/6  "RAW_Byte_1"
  in_263/1 -> RTICANMMCaptureMessage_20/7  "RAW_Byte_2"
  in_264/1 -> RTICANMMCaptureMessage_20/8  "RAW_Byte_3"
  in_265/1 -> RTICANMMCaptureMessage_20/9  "RAW_Byte_4"
  in_266/1 -> RTICANMMCaptureMessage_20/10  "RAW_Byte_5"
  in_267/1 -> RTICANMMCaptureMessage_20/11  "RAW_Byte_6"
  in_268/1 -> RTICANMMCaptureMessage_20/12  "RAW_Byte_7"
  in_269/1 -> RTICANMMCaptureMessage_20/13  "RAW_Byte_8"
  in_270/1 -> RTICANMMCaptureMessage_21/1  "Status"
  RTICANMMCaptureMessage_21/1 -> Mux/22  "RTICANMMCaptureMessage_21"
  in_271/1 -> RTICANMMCaptureMessage_21/2  "Time"
  in_272/1 -> RTICANMMCaptureMessage_21/3  "ID"
  in_273/1 -> RTICANMMCaptureMessage_21/4  "MessageIDFormat"
  in_274/1 -> RTICANMMCaptureMessage_21/5  "Length"
  in_275/1 -> RTICANMMCaptureMessage_21/6  "RAW_Byte_1"
  in_276/1 -> RTICANMMCaptureMessage_21/7  "RAW_Byte_2"
  in_277/1 -> RTICANMMCaptureMessage_21/8  "RAW_Byte_3"
  in_278/1 -> RTICANMMCaptureMessage_21/9  "RAW_Byte_4"
  in_279/1 -> RTICANMMCaptureMessage_21/10  "RAW_Byte_5"
  in_280/1 -> RTICANMMCaptureMessage_21/11  "RAW_Byte_6"
  in_281/1 -> RTICANMMCaptureMessage_21/12  "RAW_Byte_7"
  in_282/1 -> RTICANMMCaptureMessage_21/13  "RAW_Byte_8"
  in_283/1 -> RTICANMMCaptureMessage_22/1  "Status"
  RTICANMMCaptureMessage_22/1 -> Mux/23  "RTICANMMCaptureMessage_22"
  in_284/1 -> RTICANMMCaptureMessage_22/2  "Time"
  in_285/1 -> RTICANMMCaptureMessage_22/3  "ID"
  in_286/1 -> RTICANMMCaptureMessage_22/4  "MessageIDFormat"
  in_287/1 -> RTICANMMCaptureMessage_22/5  "Length"
  in_288/1 -> RTICANMMCaptureMessage_22/6  "RAW_Byte_1"
  in_289/1 -> RTICANMMCaptureMessage_22/7  "RAW_Byte_2"
  in_290/1 -> RTICANMMCaptureMessage_22/8  "RAW_Byte_3"
  in_291/1 -> RTICANMMCaptureMessage_22/9  "RAW_Byte_4"
  in_292/1 -> RTICANMMCaptureMessage_22/10  "RAW_Byte_5"
  in_293/1 -> RTICANMMCaptureMessage_22/11  "RAW_Byte_6"
  in_294/1 -> RTICANMMCaptureMessage_22/12  "RAW_Byte_7"
  in_295/1 -> RTICANMMCaptureMessage_22/13  "RAW_Byte_8"
  in_296/1 -> RTICANMMCaptureMessage_23/1  "Status"
  RTICANMMCaptureMessage_23/1 -> Mux/24  "RTICANMMCaptureMessage_23"
  in_297/1 -> RTICANMMCaptureMessage_23/2  "Time"
  in_298/1 -> RTICANMMCaptureMessage_23/3  "ID"
  in_299/1 -> RTICANMMCaptureMessage_23/4  "MessageIDFormat"
  in_300/1 -> RTICANMMCaptureMessage_23/5  "Length"
  in_301/1 -> RTICANMMCaptureMessage_23/6  "RAW_Byte_1"
  in_302/1 -> RTICANMMCaptureMessage_23/7  "RAW_Byte_2"
  in_303/1 -> RTICANMMCaptureMessage_23/8  "RAW_Byte_3"
  in_304/1 -> RTICANMMCaptureMessage_23/9  "RAW_Byte_4"
  in_305/1 -> RTICANMMCaptureMessage_23/10  "RAW_Byte_5"
  in_306/1 -> RTICANMMCaptureMessage_23/11  "RAW_Byte_6"
  in_307/1 -> RTICANMMCaptureMessage_23/12  "RAW_Byte_7"
  in_308/1 -> RTICANMMCaptureMessage_23/13  "RAW_Byte_8"
  in_309/1 -> RTICANMMCaptureMessage_24/1  "Status"
  RTICANMMCaptureMessage_24/1 -> Mux/25  "RTICANMMCaptureMessage_24"
  in_310/1 -> RTICANMMCaptureMessage_24/2  "Time"
  in_311/1 -> RTICANMMCaptureMessage_24/3  "ID"
  in_312/1 -> RTICANMMCaptureMessage_24/4  "MessageIDFormat"
  in_313/1 -> RTICANMMCaptureMessage_24/5  "Length"
  in_314/1 -> RTICANMMCaptureMessage_24/6  "RAW_Byte_1"
  in_315/1 -> RTICANMMCaptureMessage_24/7  "RAW_Byte_2"
  in_316/1 -> RTICANMMCaptureMessage_24/8  "RAW_Byte_3"
  in_317/1 -> RTICANMMCaptureMessage_24/9  "RAW_Byte_4"
  in_318/1 -> RTICANMMCaptureMessage_24/10  "RAW_Byte_5"
  in_319/1 -> RTICANMMCaptureMessage_24/11  "RAW_Byte_6"
  in_320/1 -> RTICANMMCaptureMessage_24/12  "RAW_Byte_7"
  in_321/1 -> RTICANMMCaptureMessage_24/13  "RAW_Byte_8"
  in_322/1 -> RTICANMMCaptureMessage_25/1  "Status"
  RTICANMMCaptureMessage_25/1 -> Mux/26  "RTICANMMCaptureMessage_25"
  in_323/1 -> RTICANMMCaptureMessage_25/2  "Time"
  in_324/1 -> RTICANMMCaptureMessage_25/3  "ID"
  in_325/1 -> RTICANMMCaptureMessage_25/4  "MessageIDFormat"
  in_326/1 -> RTICANMMCaptureMessage_25/5  "Length"
  in_327/1 -> RTICANMMCaptureMessage_25/6  "RAW_Byte_1"
  in_328/1 -> RTICANMMCaptureMessage_25/7  "RAW_Byte_2"
  in_329/1 -> RTICANMMCaptureMessage_25/8  "RAW_Byte_3"
  in_330/1 -> RTICANMMCaptureMessage_25/9  "RAW_Byte_4"
  in_331/1 -> RTICANMMCaptureMessage_25/10  "RAW_Byte_5"
  in_332/1 -> RTICANMMCaptureMessage_25/11  "RAW_Byte_6"
  in_333/1 -> RTICANMMCaptureMessage_25/12  "RAW_Byte_7"
  in_334/1 -> RTICANMMCaptureMessage_25/13  "RAW_Byte_8"
  Mux/1 -> out/1

== system hcu_main_dspace/RTICANMM MainBlock1/ModelClose ==
